simulink model "Mpu_AxModel"  (R2015b)
settings: Solver=ode5  StartTime=0.0  StopTime=180  FixedStep=1/mpu_sampling_frequency  RelTol=1e-3
values from neighbouring files (symbols this model uses):
  mpu_ax_bias = mean(Accel_X)    [mpu_ax.m]
  mpu_ax_noise_density = 300e-6    (= 0.0003)    [imu_settings.m]    (also in mpu_ax.m)
  mpu_ax_sensitivity = 1/16384    (= 6.103515625e-05)    [imu_settings.m]    (also in mpu_ax.m)
  mpu_ax_w = 460    [imu_settings.m]    (also in mpu_ax.m)
  mpu_sampling_frequency = 819.2    [adis_imu_settings.m]    (also in imu_settings.m = 200; mpu_plot.m = 200)
undefined symbols (not defined in the file or in its folder): w_ax, wn_ax, zeta_ax
libraries: simulink x1
settings Model: Creator=TOOsab  LastModifiedBy=TOOsab

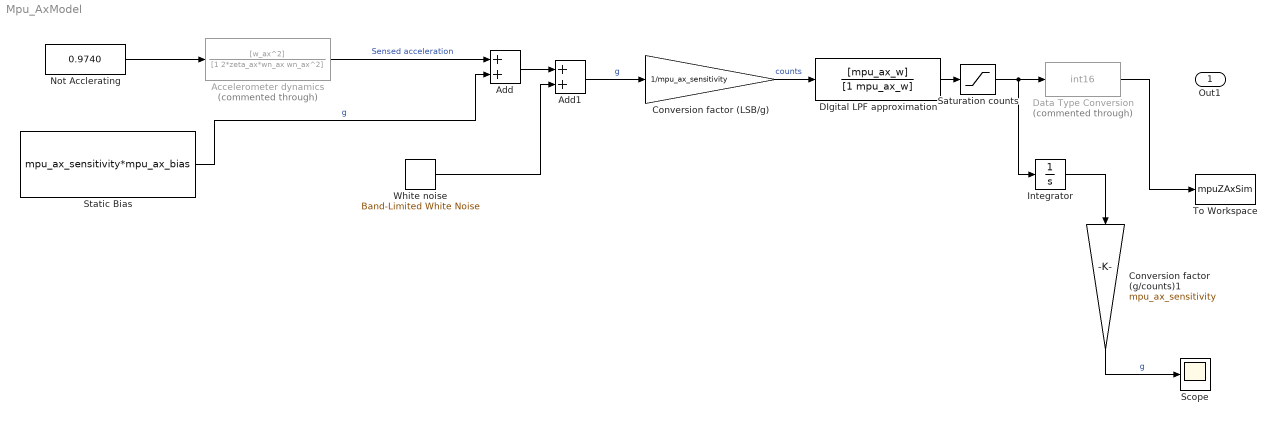
== system Mpu_AxModel ==
  Accelerometer dynamics : TransferFcn  Commented=through  Numerator=[w_ax^2]  Denominator=[1 2*zeta_ax*wn_ax wn_ax^2]
  Add : Sum
  Add1 : Sum
  Conversion factor (LSB/g) : Gain  Gain=1/mpu_ax_sensitivity
  Conversion factor (g/counts)1 : Gain  Gain=mpu_ax_sensitivity
  DIgital LPF approximation : TransferFcn  Numerator=[mpu_ax_w]  Denominator=[1 mpu_ax_w]
  Data Type Conversion : DataTypeConversion  Commented=through  OutDataTypeStr=int16
  Integrator : Integrator
  "Not Acclerating " : Constant  Value=0.9740
  "Saturation counts " : Saturate  UpperLimit=2^15  LowerLimit=-2^15
  Scope : Scope
  Static Bias : Constant  Value=mpu_ax_sensitivity*mpu_ax_bias
  To Workspace : ToWorkspace  VariableName=mpuZAxSim  SampleTime=-1
  White noise : simulink/Sources/Band-Limited White Noise  Cov=[(mpu_ax_noise_density)^2]  Ts=1/mpu_sampling_frequency  seed=[23341]
  Out1 : Outport
  wires:
  Conversion factor (LSB/g)/1 -> DIgital LPF approximation/1  "counts"
  Static Bias/1 -> Add/2  "g"
  Accelerometer dynamics/1 -> Add/1  "Sensed acceleration"
  White noise/1 -> Add1/2
  Add/1 -> Add1/1
  Add1/1 -> Conversion factor (LSB/g)/1  "g"
  DIgital LPF approximation/1 -> "Saturation counts "/1
  "Saturation counts "/1 -> Integrator/1, Data Type Conversion/1
  Data Type Conversion/1 -> To Workspace/1
  "Not Acclerating "/1 -> Accelerometer dynamics/1
  Integrator/1 -> Conversion factor (g/counts)1/1
  Conversion factor (g/counts)1/1 -> Scope/1  "g"
